simulink model "StairCaseWaveGeneration"  (R2020b)
settings: Solver=VariableStepAuto  StartTime=0.0  StopTime=1  FixedStep=1  MaxStep=0.01  RelTol=1e-3
settings Model: Creator=99003736  LastModifiedBy=99003736

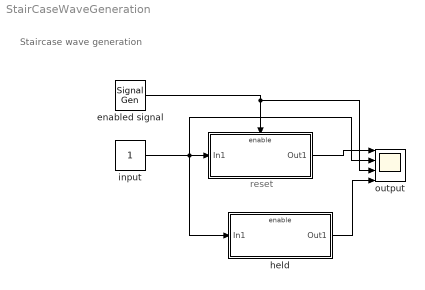
== system StairCaseWaveGeneration ==
  note: reset
  note: Staircase wave generation
  " " : Subsystem  TreatAsAtomicUnit=on
  " held" : Subsystem  TreatAsAtomicUnit=on
  enabled signal : SignalGenerator  WaveForm=square  Frequency=3
  input : Constant
  output : Scope  NumInputPorts=4
  wires:
  input/1 -> " held"/1(In1), output/2, " "/1(In1)
  " "/1(Out1) -> output/1
  enabled signal/1 -> output/3, " "/Enable
  " held"/1(Out1) -> output/4

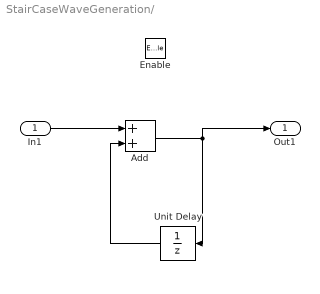
== system StairCaseWaveGeneration/  ==
  In1 : Inport
  Enable : EnablePort  StatesWhenEnabling=reset
  Add : Sum
  Unit Delay : UnitDelay  SampleTime=-1  HasFrameUpgradeWarning=on
  Out1 : Outport
  wires:
  Unit Delay/1 -> Add/2
  Add/1 -> Out1/1, Unit Delay/1
  In1/1 -> Add/1

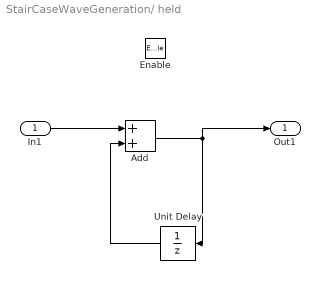
== system StairCaseWaveGeneration/ held ==
  In1 : Inport
  Enable : EnablePort
  Add : Sum
  Unit Delay : UnitDelay  SampleTime=-1  HasFrameUpgradeWarning=on
  Out1 : Outport
  wires:
  Unit Delay/1 -> Add/2
  Add/1 -> Out1/1, Unit Delay/1
  In1/1 -> Add/1
